simulink model "UDP_Test"  (R2019b)
settings: Solver=VariableStepAuto  StartTime=0.0  StopTime=10.0  RelTol=1e-3
undefined symbols (not defined in the file): __PRM__SERIALIZED__DATA__, SubsystemReferenceBlock
settings Model: Creator=toons  LastModifiedBy=toons

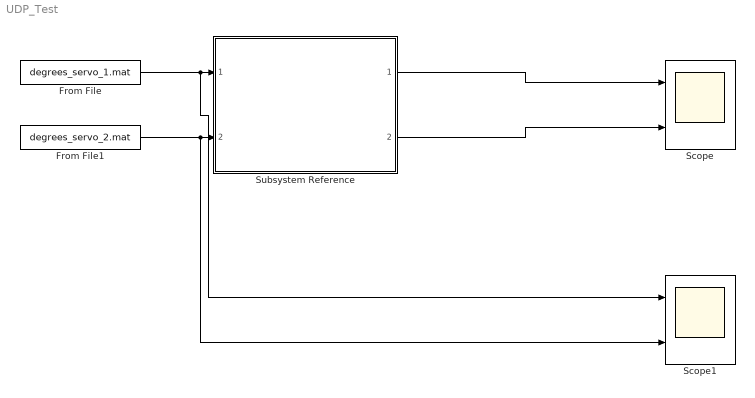
== system UDP_Test ==
  From File : FromFile  FileName=degrees_servo_1.mat  SampleTime=0.01
  From File1 : FromFile  FileName=degrees_servo_2.mat  SampleTime=0.01
  Scope : Scope  NumInputPorts=2
  Scope1 : Scope  NumInputPorts=2
  Subsystem Reference : Subsystem  BlockKeywords=__PRM__SERIALIZED__DATA__:SubsystemReferenceBlock  ReferencedSubsystem=UDP_MCU
  wires:
  From File/1 -> Scope1/1, Subsystem Reference/1
  From File1/1 -> Scope1/2, Subsystem Reference/2
  Subsystem Reference/1 -> Scope/1
  Subsystem Reference/2 -> Scope/2
